simulink model "quantizedModel"  (R2024b)
settings: Solver=FixedStepAuto  StartTime=0.0  StopTime=10.0  RelTol=1e-3
undefined symbols (not defined in the file or in its folder): qMod
libraries: dlconvfclib x5, dlactivationlib x4
settings Model: Creator=dx5entre  LastModifiedBy=dx5entre
settings OptimizationCC: DefaultParameterBehavior=Inlined  EnhancedBackFolding=on  PassReuseOutputArgsAs=Individual arguments  ZeroExternalMemoryAtStartup=off  ZeroInternalMemoryAtStartup=off  OptimizeBlockOrder=speed  DifferentSizesBufferReuse=on  OptimizationCustomize=off  EfficientTunableParamExpr=on
settings DebuggingCC: ParameterTunabilityLossMsg=error
settings SFSimCC: MATLABDynamicMemAlloc=off
settings RTWCC: Description=Embedded Coder  SystemTargetFile=ert.tlc  TemplateMakefile=ert_default_tmf
settings CodeAppCC: ForceParamTrailComments=on  IgnoreCustomStorageClasses=off  OperatorAnnotations=on  SimulinkDataObjDesc=on  SFDataObjDesc=on  InsertBlockDesc=on
settings ERTTargetCC: TargetLangStandard=C99 (ISO)  GenerateSampleERTMain=on  ERTCustomFileTemplate=example_file_process.tlc

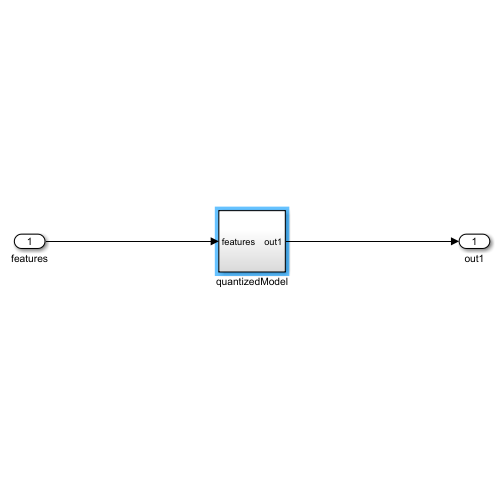
[thumbnail: Simulink's stored preview of the top-level diagram]
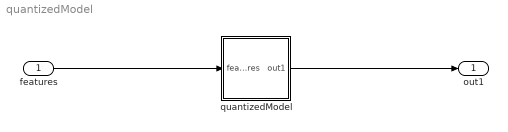
== system quantizedModel ==
  features : Inport  PortDimensions=[35]
  quantizedModel : Subsystem
  out1 : Outport
  wires:
  features/1 -> quantizedModel/1(features)
  quantizedModel/1(out1) -> out1/1

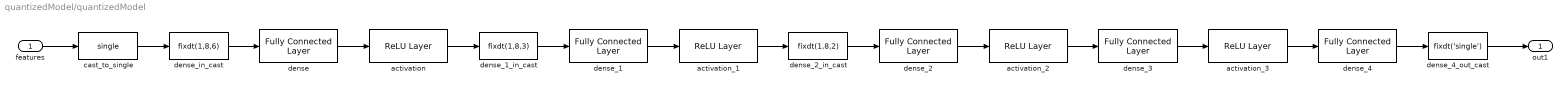
== system quantizedModel/quantizedModel ==
  features : Inport  PortDimensions=[35]
  activation : dlactivationlib/ReLU Layer  OutMin=[]  OutMax=[]  OutDataTypeStr=fixdt(1,8,1)  SampleTime=-1
  activation_1 : dlactivationlib/ReLU Layer  OutMin=[]  OutMax=[]  OutDataTypeStr=fixdt(1,8,1)  SampleTime=-1
  activation_2 : dlactivationlib/ReLU Layer  OutMin=[]  OutMax=[]  OutDataTypeStr=fixdt(1,8,3)  SampleTime=-1
  activation_3 : dlactivationlib/ReLU Layer  OutMin=[]  OutMax=[]  OutDataTypeStr=fixdt(1,8,5)  SampleTime=-1
  cast_to_single : DataTypeConversion  OutDataTypeStr=single  SaturateOnIntegerOverflow=off  RndMeth=Floor
  dense : dlconvfclib/Fully Connected Layer  Layer=qMod.Layers(2)  OutMin=[]  OutMax=[]  OutDataTypeStr=fixdt(1,8,1)  RndMeth=Nearest  SaturateOnIntegerOverflow=on  WeightsDataTypeStr=fixdt(1,8,3)  WeightsMin=[]  WeightsMax=[]  BiasDataTypeStr=fixdt(1,32,9)  BiasMin=[]  BiasMax=[]  MatrixMultiplyDataTypeStr=fixdt(1,32,9)  MatrixMultiplyMin=[]  MatrixMultiplyMax=[]  SampleTime=-1
      settings: DataFormat=C
  dense_1 : dlconvfclib/Fully Connected Layer  Layer=qMod.Layers(4)  OutMin=[]  OutMax=[]  OutDataTypeStr=fixdt(1,8,1)  RndMeth=Nearest  SaturateOnIntegerOverflow=on  WeightsDataTypeStr=fixdt(1,8,5)  WeightsMin=[]  WeightsMax=[]  BiasDataTypeStr=fixdt(1,32,8)  BiasMin=[]  BiasMax=[]  MatrixMultiplyDataTypeStr=fixdt(1,32,8)  MatrixMultiplyMin=[]  MatrixMultiplyMax=[]  SampleTime=-1
      settings: DataFormat=C
  dense_1_in_cast : DataTypeConversion  OutDataTypeStr=fixdt(1,8,3)  RndMeth=Nearest
  dense_2 : dlconvfclib/Fully Connected Layer  Layer=qMod.Layers(6)  OutMin=[]  OutMax=[]  OutDataTypeStr=fixdt(1,8,3)  RndMeth=Nearest  SaturateOnIntegerOverflow=on  WeightsDataTypeStr=fixdt(1,8,7)  WeightsMin=[]  WeightsMax=[]  BiasDataTypeStr=fixdt(1,32,9)  BiasMin=[]  BiasMax=[]  MatrixMultiplyDataTypeStr=fixdt(1,32,9)  MatrixMultiplyMin=[]  MatrixMultiplyMax=[]  SampleTime=-1
      settings: DataFormat=C
  dense_2_in_cast : DataTypeConversion  OutDataTypeStr=fixdt(1,8,2)  RndMeth=Nearest
  dense_3 : dlconvfclib/Fully Connected Layer  Layer=qMod.Layers(8)  OutMin=[]  OutMax=[]  OutDataTypeStr=fixdt(1,8,5)  RndMeth=Nearest  SaturateOnIntegerOverflow=on  WeightsDataTypeStr=fixdt(1,8,8)  WeightsMin=[]  WeightsMax=[]  BiasDataTypeStr=fixdt(1,32,11)  BiasMin=[]  BiasMax=[]  MatrixMultiplyDataTypeStr=fixdt(1,32,11)  MatrixMultiplyMin=[]  MatrixMultiplyMax=[]  SampleTime=-1
      settings: DataFormat=C
  dense_4 : dlconvfclib/Fully Connected Layer  Layer=qMod.Layers(10)  OutMin=[]  OutMax=[]  OutDataTypeStr=fixdt(1,32,13)  RndMeth=Nearest  SaturateOnIntegerOverflow=on  WeightsDataTypeStr=fixdt(1,8,8)  WeightsMin=[]  WeightsMax=[]  BiasDataTypeStr=fixdt(1,32,13)  BiasMin=[]  BiasMax=[]  MatrixMultiplyDataTypeStr=fixdt(1,32,13)  MatrixMultiplyMin=[]  MatrixMultiplyMax=[]  SampleTime=-1
      settings: DataFormat=C
  dense_4_out_cast : DataTypeConversion  OutDataTypeStr=fixdt('single')  RndMeth=Nearest
  dense_in_cast : DataTypeConversion  OutDataTypeStr=fixdt(1,8,6)  RndMeth=Nearest
  out1 : Outport
  wires:
  activation_2/1 -> dense_3/1
  cast_to_single/1 -> dense_in_cast/1
  dense_2_in_cast/1 -> dense_2/1
  dense_in_cast/1 -> dense/1
  dense_2/1 -> activation_2/1
  activation_1/1 -> dense_2_in_cast/1
  dense_4/1 -> dense_4_out_cast/1
  dense_4_out_cast/1 -> out1/1
  dense_1/1 -> activation_1/1
  features/1 -> cast_to_single/1
  dense_1_in_cast/1 -> dense_1/1
  activation_3/1 -> dense_4/1
  dense/1 -> activation/1
  dense_3/1 -> activation_3/1
  activation/1 -> dense_1_in_cast/1
